simulink model "doppler_filter"  (R2016b)
settings: Solver=FixedStepAuto  StartTime=0.0  StopTime=10^(-2)  FixedStep=10^(-10)  RelTol=1e-3  EnableMultiTasking=on
undefined symbols (not defined in the file): fdesignblkfcn, gcbh
libraries: commchan3 x1
settings Model: Creator=MOMENT OF PEACE  LastModifiedBy=MOMENT OF PEACE
settings DataIOCC: LimitDataPoints=on  SaveFormat=Array
settings OptimizationCC: LifeSpan=inf
settings DebuggingCC: AllowSymbolicDim=off  SFUnexpectedBacktrackingDiag=warning  SFNoUnconditionalDefaultTransitionDiag=warning  SFExecutionAtInitializationDiag=none
settings HardwareCC: ProdBitPerPointer=32  ProdBitPerSizeT=32  ProdBitPerPtrDiffT=32  ProdLargestAtomicFloat=None  ProdIntDivRoundTo=Undefined  ProdEndianess=Unspecified  ProdWordSize=32  ProdHWDeviceType=32-bit Generic
settings ModelReferenceCC: PropagateSignalLabelsOutOfModel=off
settings GRTTargetCC: TargetLangStandard=C89/C90 (ANSI)  GeneratePreprocessorConditionals=Disable all
settings ConfigComp: CovMetricSettings=dw  CovHtmlReporting=on  CovSaveCumulativeToWorkspaceVar=on  CovSaveSingleToWorkspaceVar=on  CovExternalEMLEnable=off

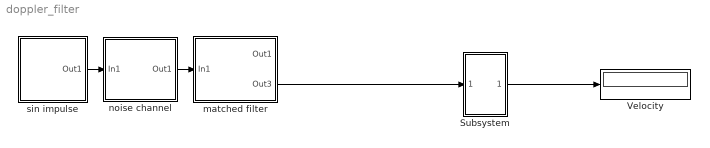
== system doppler_filter ==
  Subsystem : Subsystem
  Velocity : Display
  matched filter : Subsystem
  noise channel : Subsystem
  sin impulse : Subsystem  mask{v=20}
      mask prompts: v "velocity"
      mask init:
      | fd = 2*v/0.3;
      | f = (1e9 + fd)*2*pi
  wires:
  noise channel/1(Out1) -> matched filter/1(In1)
  sin impulse/1(Out1) -> noise channel/1(In1)
  matched filter/2(Out3) -> Subsystem/1(In1)
  Subsystem/1(Out1) -> Velocity/1

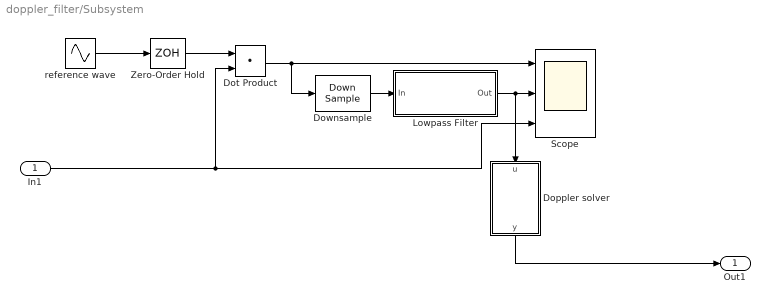
== system doppler_filter/Subsystem ==
  In1 : Inport
  Doppler solver : MATLAB Function  TreatAsAtomicUnit=on
  Dot Product : DotProduct  InputSameDT=on  OutDataTypeStr=Inherit: Inherit via internal rule
  Downsample : DownSample  N=300000  phase=104
  Lowpass Filter : Subsystem  DialogController=fdesignblkfcn  InitFcn=fdesignblkfcn(gcbh, {'InitFcn'});  mask(Lowpass Filter){}
      mask help: Design a lowpass filter
      settings: CopyFcn=fdesignblkfcn(gcbh, {'CopyFcn'});
      mask Help: helpview(mapfilelocation('dsp'), 'dsplowpassfilter');
      mask Display: disp('Lowpass')
  Scope : Scope  NumInputPorts=3
  Zero-Order Hold : ZeroOrderHold  SampleTime=10^(-10)
  reference wave : Sin  Frequency=1000000000*2*pi  SampleTime=0
  Out1 : Outport
  wires:
  reference wave/1 -> Zero-Order Hold/1
  Downsample/1 -> Lowpass Filter/1(In)
  Dot Product/1 -> Scope/1, Downsample/1
  Zero-Order Hold/1 -> Dot Product/1
  In1/1 -> Scope/3, Dot Product/2
  Doppler solver/1(y) -> Out1/1
  Lowpass Filter/1(Out) -> Scope/2, Doppler solver/1(u)

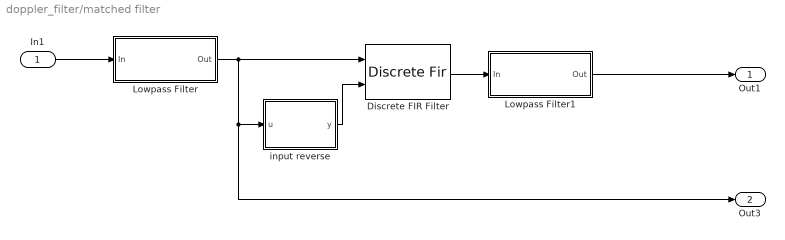
== system doppler_filter/matched filter ==
  In1 : Inport
  Discrete FIR Filter : DiscreteFir  CoefSource=Input port  Coefficients=[1 1 1 1 1 1]  InputProcessing=Columns as channels (frame based)
      settings: InputPortMap=u0,u1
  Lowpass Filter : Subsystem  DialogController=fdesignblkfcn  InitFcn=fdesignblkfcn(gcbh, {'InitFcn'});  mask(Lowpass Filter){}
      mask help: Design a lowpass filter
      settings: CopyFcn=fdesignblkfcn(gcbh, {'CopyFcn'});
      mask Help: helpview(mapfilelocation('dsp'), 'dsplowpassfilter');
      mask Display: disp('Lowpass')
  Lowpass Filter1 : Subsystem  DialogController=fdesignblkfcn  InitFcn=fdesignblkfcn(gcbh, {'InitFcn'});  mask(Lowpass Filter){}
      mask help: Design a lowpass filter
      settings: CopyFcn=fdesignblkfcn(gcbh, {'CopyFcn'});
      mask Help: helpview(mapfilelocation('dsp'), 'dsplowpassfilter');
      mask Display: disp('Lowpass')
  input reverse : MATLAB Function  TreatAsAtomicUnit=on
  Out1 : Outport
  Out3 : Outport  Port=2
  wires:
  In1/1 -> Lowpass Filter/1(In)
  input reverse/1(y) -> Discrete FIR Filter/2
  Discrete FIR Filter/1 -> Lowpass Filter1/1(In)
  Lowpass Filter/1(Out) -> Discrete FIR Filter/1, Out3/1, input reverse/1(u)
  Lowpass Filter1/1(Out) -> Out1/1

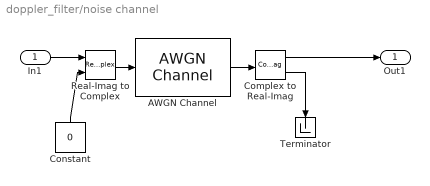
== system doppler_filter/noise channel ==
  In1 : Inport
  AWGN Channel : commchan3/AWGN Channel  InputProcessing=Columns as channels (frame based)  seed=67  noiseMode="Signal to noise ratio  (SNR)"  EbNodB=10  EsNodB=10  SNRdB=15  bitsPerSym=1  Ps=1  Tsym=1  variance=1
  Complex to Real-Imag : ComplexToRealImag
  Constant : Constant  Value=0
  Real-Imag to Complex : RealImagToComplex
  Terminator : Terminator
  Out1 : Outport
  wires:
  Real-Imag to Complex/1 -> AWGN Channel/1
  Constant/1 -> Real-Imag to Complex/2
  Complex to Real-Imag/2 -> Terminator/1
  In1/1 -> Real-Imag to Complex/1
  AWGN Channel/1 -> Complex to Real-Imag/1
  Complex to Real-Imag/1 -> Out1/1

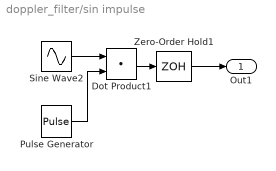
== system doppler_filter/sin impulse ==
  Dot Product1 : DotProduct  InputSameDT=on  OutDataTypeStr=Inherit: Inherit via internal rule
  Pulse Generator : DiscretePulseGenerator  Period=3000  PulseWidth=100  SampleTime=10^(-10)
  Sine Wave2 : Sin  Frequency=f  Phase=0.3*pi  SampleTime=0
  Zero-Order Hold1 : ZeroOrderHold  SampleTime=10^(-10)
  Out1 : Outport
  wires:
  Dot Product1/1 -> Zero-Order Hold1/1
  Pulse Generator/1 -> Dot Product1/2
  Zero-Order Hold1/1 -> Out1/1
  Sine Wave2/1 -> Dot Product1/1

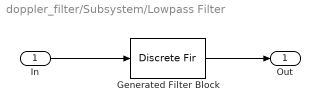
== system doppler_filter/Subsystem/Lowpass Filter ==
  In : Inport
  Generated Filter Block : DiscreteFir  Tag=BlockMethodSubSystem  Coefficients=[0.00444194733209979115 0.0054220324433853391 -0.0118651041659676611 -0.0311692725865293438 -0.00867203647139627026 0.0390340643789495317 0.0194541464420488128 -0.0723156718204192722 -0.0634598005717867258 0.164988409771359118 0.428191589429428698 0.428191589429428698 0.164988409771359118 -0.0634598005717867258 -0.0723156718204192722 0.0194541464420488128 0.0390340643789495317 -0.00867203647139627026 -0.0311692725865293438 -0.0118651041659676611 0.0054220324433853391 0.00444194733209979115]  InputProcessing=Columns as channels (frame based)
  Out : Outport
  wires:
  In/1 -> Generated Filter Block/1
  Generated Filter Block/1 -> Out/1

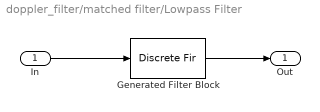
== system doppler_filter/matched filter/Lowpass Filter ==
  In : Inport
  Generated Filter Block : DiscreteFir  Tag=BlockMethodSubSystem  Coefficients=[-0.00882242952209379323 -0.00250396131135136295 0.0203488178406029327 0.00845153638179320724 -0.00156508516764006927 0.0105860024294243335 -0.00352454868452364151 0.00077576045905514146 0.00717622040828255932 -0.00940111963814425564 0.00797382618152611515 -0.000273978864866431318 -0.00850196312346529828 0.0141906978084733945 -0.0119506479715848612 0.00181855656901186435 0.0118184144727089858 -0.0210959922579116305 0.0193002857308069292 -0.00470681791085527865 -0.0167959060315205945 0.0337033448793372867 -0.0339636229705798098 0.0118324414990105195 0.0272315640460091407 -0.0660974718487657292 0.0800981455589089425 -0.0421164040979259552 -0.0871991530250003505 0.590547367711231064 0.590547367711231064 -0.0871991530250003505 -0.0421164040979259552 0.0800981455589089425 -0.0660974718487657292 0.0272315640460091407 0.0118324414990105195 -0.0339636229705798098 0.0337033448793372867 -0.0167959060315205945 -0.00470681791085527865 0.0193002857308069292 -0.0210959922579116305 0.0118184144727089858 0.00181855656901186435 -0.0119506479715848612 0.0141906978084733945 -0.00850196312346529828 -0.000273978864866431318 0.00797382618152611515 -0.00940111963814425564 0.00717622040828255932 0.00077576045905514146 -0.00352454868452364151 0.0105860024294243335 -0.00156508516764006927 0.00845153638179320724 0.0203488178406029327 -0.00250396131135136295 -0.00882242952209379323]  InputProcessing=Columns as channels (frame based)
  Out : Outport
  wires:
  In/1 -> Generated Filter Block/1
  Generated Filter Block/1 -> Out/1

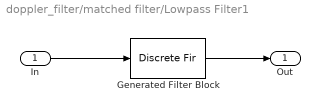
== system doppler_filter/matched filter/Lowpass Filter1 ==
  In : Inport
  Generated Filter Block : DiscreteFir  Tag=BlockMethodSubSystem  Coefficients=[-0.00882242952209379323 -0.00250396131135136295 0.0203488178406029327 0.00845153638179320724 -0.00156508516764006927 0.0105860024294243335 -0.00352454868452364151 0.00077576045905514146 0.00717622040828255932 -0.00940111963814425564 0.00797382618152611515 -0.000273978864866431318 -0.00850196312346529828 0.0141906978084733945 -0.0119506479715848612 0.00181855656901186435 0.0118184144727089858 -0.0210959922579116305 0.0193002857308069292 -0.00470681791085527865 -0.0167959060315205945 0.0337033448793372867 -0.0339636229705798098 0.0118324414990105195 0.0272315640460091407 -0.0660974718487657292 0.0800981455589089425 -0.0421164040979259552 -0.0871991530250003505 0.590547367711231064 0.590547367711231064 -0.0871991530250003505 -0.0421164040979259552 0.0800981455589089425 -0.0660974718487657292 0.0272315640460091407 0.0118324414990105195 -0.0339636229705798098 0.0337033448793372867 -0.0167959060315205945 -0.00470681791085527865 0.0193002857308069292 -0.0210959922579116305 0.0118184144727089858 0.00181855656901186435 -0.0119506479715848612 0.0141906978084733945 -0.00850196312346529828 -0.000273978864866431318 0.00797382618152611515 -0.00940111963814425564 0.00717622040828255932 0.00077576045905514146 -0.00352454868452364151 0.0105860024294243335 -0.00156508516764006927 0.00845153638179320724 0.0203488178406029327 -0.00250396131135136295 -0.00882242952209379323]  InputProcessing=Columns as channels (frame based)
  Out : Outport
  wires:
  Generated Filter Block/1 -> Out/1
  In/1 -> Generated Filter Block/1

== matlab function doppler_filter/Subsystem/Doppler solver ==
  data: u input; y output
function y = fcn(u)
%#codegen
persistent sum;
persistent pre;
persistent v;

if isempty(sum)
    sum = 0;
end

if isempty(pre)
    pre = 0;
end

if isempty(v)
    v = 0;
end

x = u * pre;
pre = u;

if x > 0
    sum = sum + 1;
else
    vtemp = 3e9/(4*sum);
    if vtemp < 150
        v = vtemp;
    end
    sum = 0;
end

y = v;

== matlab function doppler_filter/matched filter/input reverse ==
  data: u input; y output
function y = fcn(u)
%#codegen

y = u(end:-1:1);
